simulink model "model"  (R2018a)
settings: Solver=VariableStepAuto  StartTime=0.0  StopTime=model_time  MaxStep=0.01  RelTol=1e-3
values from neighbouring files (symbols this model uses):
  a0 = -g/h    (= -15.0923076923)    [init.m]
  b0 = V^2/(h*c)    (= 32.0512820513)    [init.m]
  b1 = (l*V)/(h*c)    (= 1.60256410256)    [init.m]
  const_sourse = 0.1    [init.m]
  K = 0.001    [init.m]
libraries: simulink_extras x2
settings Model: Creator=Asus  LastModifiedBy=Asus

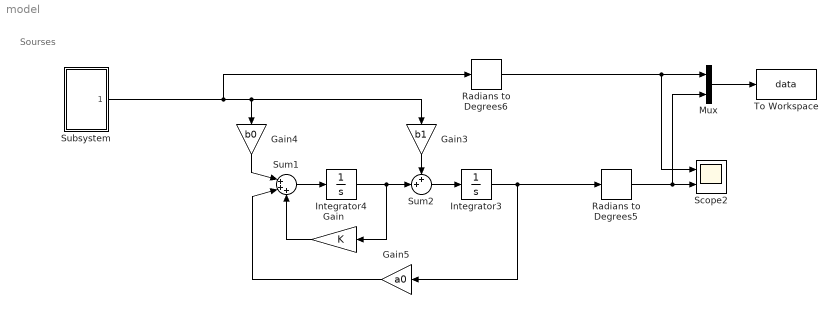
== system model ==
  note: Sourses
  Gain : Gain  Gain=K
  Gain3 : Gain  Gain=b1
  Gain4 : Gain  Gain=b0
  Gain5 : Gain  Gain=a0
  Integrator3 : Integrator
  Integrator4 : Integrator
  Mux : Mux  Inputs=2
  Radians to Degrees5 : simulink_extras/Transformations/Radians to Degrees
  Radians to Degrees6 : simulink_extras/Transformations/Radians to Degrees
  Scope2 : Scope  NumInputPorts=2
  Subsystem : Subsystem
  Sum1 : Sum  Inputs=|+++
  Sum2 : Sum  Inputs=++|
  To Workspace : ToWorkspace  VariableName=data  SampleTime=-1
  wires:
  Sum1/1 -> Integrator4/1
  Gain4/1 -> Sum1/1
  Integrator4/1 -> Gain/1, Sum2/2
  Sum2/1 -> Integrator3/1
  Gain3/1 -> Sum2/1
  Integrator3/1 -> Gain5/1, Radians to Degrees5/1
  Radians to Degrees6/1 -> Mux/1, Scope2/1
  Gain5/1 -> Sum1/2
  Gain/1 -> Sum1/3
  Mux/1 -> To Workspace/1
  Radians to Degrees5/1 -> Mux/2, Scope2/2
  Subsystem/1(sourses) -> Radians to Degrees6/1, Gain3/1, Gain4/1

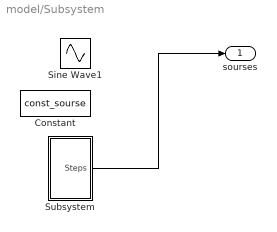
== system model/Subsystem ==
  Constant : Constant  Value=const_sourse
  Sine Wave1 : Sin  Amplitude=0.3  Frequency=0.1  SampleTime=0
  Subsystem : Subsystem
  sourses : Outport
  wires:
  Subsystem/1(Steps) -> sourses/1

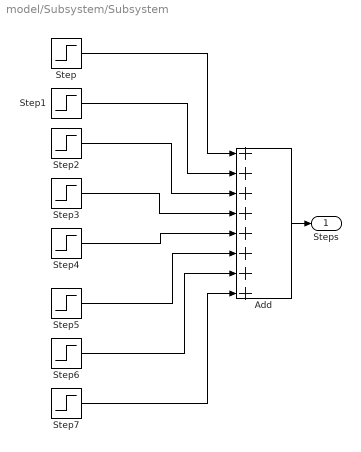
== system model/Subsystem/Subsystem ==
  Add : Sum  Inputs=++++++++
  Step : Step  After=0.1  SampleTime=0
  Step1 : Step  Time=2  After=-0.2  SampleTime=0
  Step2 : Step  Time=4  After=0.15  SampleTime=0
  Step3 : Step  Time=5  After=-0.05  SampleTime=0
  Step4 : Step  Time=7  After=0.1  SampleTime=0
  Step5 : Step  Time=9  After=-0.15  SampleTime=0
  Step6 : Step  Time=10  After=0.025  SampleTime=0
  Step7 : Step  Time=11  After=0.025  SampleTime=0
  Steps : Outport
  wires:
  Step7/1 -> Add/8
  Step1/1 -> Add/2
  Add/1 -> Steps/1
  Step/1 -> Add/1
  Step2/1 -> Add/3
  Step4/1 -> Add/5
  Step3/1 -> Add/4
  Step6/1 -> Add/7
  Step5/1 -> Add/6
